simulink model "Golbal_to_Local_TrafficObject"  (R2022b)
settings: Solver=VariableStepAuto  StartTime=0.0  StopTime=10.0  RelTol=1e-3
settings Model: Creator=USER  LastModifiedBy=USER

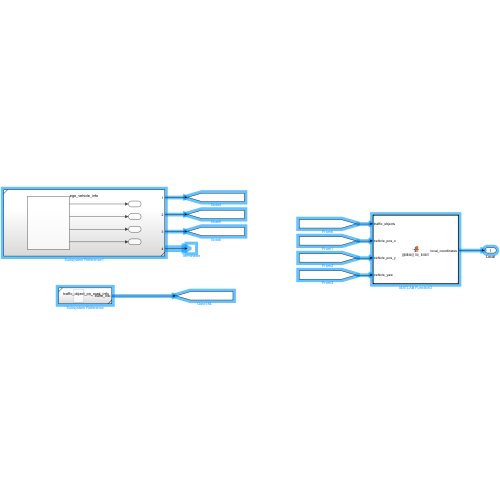
[thumbnail: Simulink's stored preview of the top-level diagram]
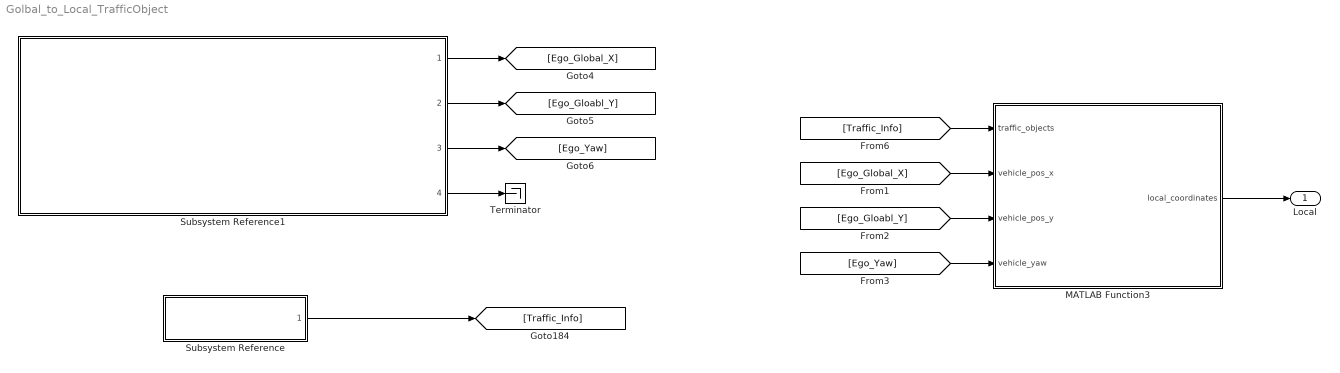
== system Golbal_to_Local_TrafficObject ==
  MATLAB Function3 : MATLAB Function  TreatAsAtomicUnit=on
  Subsystem Reference : Subsystem  ReferencedSubsystem=traffic_object_on_road_info
  Subsystem Reference1 : Subsystem  ReferencedSubsystem=ego_vehicle_info
  Terminator : Terminator
  Local : Outport
  wires:
  [Ego_Gloabl_Y] -> MATLAB Function3/3(vehicle_pos_y)
  [Ego_Global_X] -> MATLAB Function3/2(vehicle_pos_x)
  [Ego_Yaw] -> MATLAB Function3/4(vehicle_yaw)
  [Traffic_Info] -> MATLAB Function3/1(traffic_objects)
  Subsystem Reference1/2 -> [Ego_Gloabl_Y]
  Subsystem Reference1/1 -> [Ego_Global_X]
  MATLAB Function3/1(local_coordinates) -> Local/1
  Subsystem Reference1/3 -> [Ego_Yaw]
  Subsystem Reference/1 -> [Traffic_Info]
  Subsystem Reference1/4 -> Terminator/1

== matlab function Golbal_to_Local_TrafficObject/MATLAB Function3 ==
  settings: updateMethod=DISCRETE  sampleTime=0.05
  data: local_coordinates output size=[30, 2]; traffic_objects input; vehicle_pos_x input; vehicle_pos_y input; vehicle_yaw input
function local_coordinates = global_to_local(traffic_objects, vehicle_pos_x, vehicle_pos_y, vehicle_yaw)
    % 차량 위치를 기준으로 변환 (평행 이동)
    delta_x = traffic_objects(:,1) - vehicle_pos_x;
    delta_y = traffic_objects(:,2) - vehicle_pos_y;
    

    % 차량의 요(방향)에 따른 회전 변환
    x_l = cos(vehicle_yaw) * delta_x + sin(vehicle_yaw) * delta_y;
    y_l = -sin(vehicle_yaw) * delta_x + cos(vehicle_yaw) * delta_y;
    
    coder.varsize('local_coordinates', [30, 2]);
    local_coordinates = zeros(size(traffic_objects,1),2); % 지역 좌표를 저장할 배열
    local_coordinates = horzcat(x_l,y_l);
end
